simulink model "FCS-MPTC_10VVPTC_OEW_Simulink_file"  (R2024a)
settings: Solver=ode5  StartTime=0.0  StopTime=2  FixedStep=Ts  RelTol=1e-3
values from neighbouring files (symbols this model uses):
  J = 0.0148    [FivePhasePTCOEW.m]
  Ki = 0.0022    [FivePhasePTCOEW.m]
  Kp = 0.032    [FivePhasePTCOEW.m]
  kr = Lm/Lr    (= 0.941444444444)    [FivePhasePTCOEW.m]
  Lls = 6e-3    (= 0.006)    [FivePhasePTCOEW.m]
  Lm = 84.73e-3    (= 0.08473)    [FivePhasePTCOEW.m]
  p = 2    [FivePhasePTCOEW.m]
  r_sigma = Rs+kr^2*Rr    (= 2.3085710516)    [FivePhasePTCOEW.m]
  Rs = 1.05    [FivePhasePTCOEW.m]
  sf_nom = 0.2    [FivePhasePTCOEW.m]
  T_nom = 5    [FivePhasePTCOEW.m]
  t_sigma = sigma*Ls/r_sigma    (= 0.0044319243348)    [FivePhasePTCOEW.m]
  tr = Lr/Rr    (= 0.0633802816901)    [FivePhasePTCOEW.m]
  Ts = 5e-5    (= 5e-05)    [FivePhasePTCOEW.m]
  Vdc = 100    [FivePhasePTCOEW.m]
undefined symbols (not defined in the file or in its folder): DiscIntNeverNeededParam, j
libraries: simulink x2, simulink_extras x1, spspowerguiLib x1
settings Model: Creator=NARESH  LastModifiedBy=USER
settings ModelReferenceCC: EnableRefExpFcnMdlSchedulingChecks=on
settings RTWCC: GPUComputeCapability=3.5

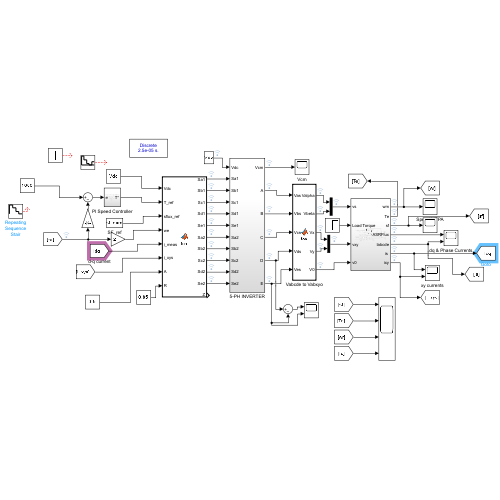
[thumbnail: Simulink's stored preview of the top-level diagram]
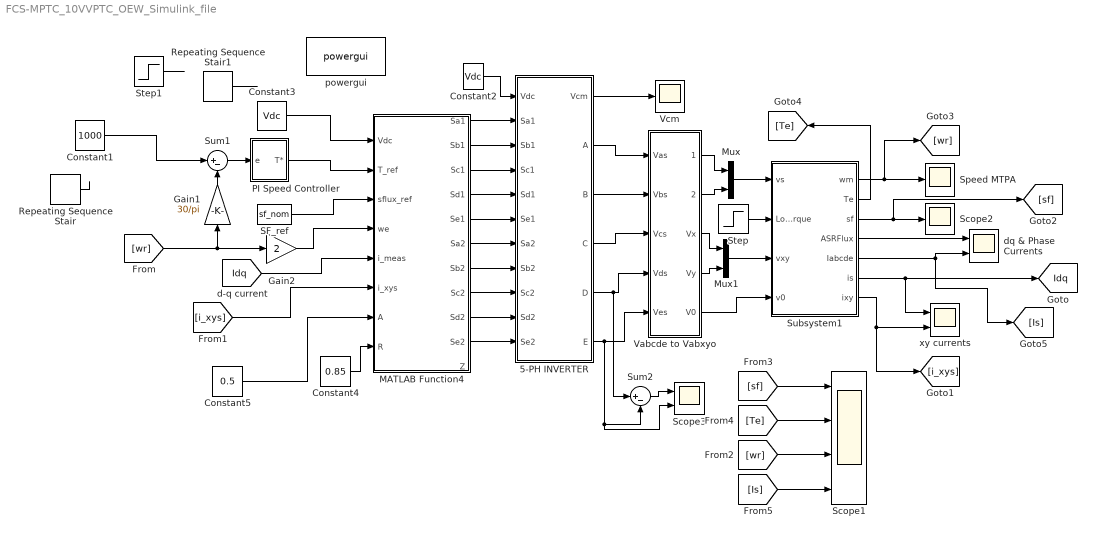
== system FCS-MPTC_10VVPTC_OEW_Simulink_file ==
  5-PH INVERTER : Subsystem
  Constant1 : Constant  Value=1000  SampleTime=Ts
  Constant2 : Constant  Value=Vdc  SampleTime=Ts
  Constant3 : Constant  Value=Vdc  SampleTime=Ts
  Constant4 : Constant  Value=0.85  SampleTime=Ts
  Constant5 : Constant  Value=0.5  SampleTime=Ts
  Gain1 : Gain  Gain=30/pi
  Gain2 : Gain  Gain=2
  MATLAB Function4 : MATLAB Function  TreatAsAtomicUnit=on
  Mux : Mux  Inputs=2
  Mux1 : Mux  Inputs=2
  PI Speed Controller : Subsystem
  Repeating Sequence Stair : simulink/Sources/Repeating Sequence Stair  OutValues=[1400 1000 500 200 ].'  tsamp=1.5  OutMin=[]  OutMax=[]  OutDataTypeStr=double  OutputDataTypeScalingMode=double  OutDataType=fixdt(0,8)  ConRadixGroup=Best Precision: Vector-wise  OutScaling=2^-12
  Repeating Sequence Stair1 : simulink/Sources/Repeating Sequence Stair  OutValues=[1400 800 200 0 500]  tsamp=1  OutMin=[]  OutMax=[]  OutDataTypeStr=double  OutputDataTypeScalingMode=double  OutDataType=fixdt(0,8)  ConRadixGroup=Best Precision: Vector-wise  OutScaling=2^-12
  SF_ref : Constant  Value=sf_nom  SampleTime=Ts
  Scope1 : Scope  NumInputPorts=4
  Scope2 : Scope
  Scope3 : Scope  NumInputPorts=2
  Speed MTPA : Scope
  Step : Step  After=0  SampleTime=0
  Step1 : Step  Before=400  After=-400  SampleTime=Ts
  Subsystem1 : Subsystem
  Sum1 : Sum  Inputs=|+-
  Sum2 : Sum  Inputs=|+-
  Vabcde to Vabxyo : MATLAB Function  TreatAsAtomicUnit=on
  Vcm : Scope
  dq & Phase Currents : Scope  NumInputPorts=2
  powergui : spspowerguiLib/powergui  Priority=1  SimulationMode=Discrete  SampleTime=Ts  frequency=60  Iterations=50  frequencyindice=60  Pbase=100e6  ErrMax=1e-4  UnitsV=kV  UnitsW=MW  buscounter=0  FunctionMessages=off  echomessages=off  EnableUseOfTLC=off  CurrentSourceSwitches=off  DisableSnubberDevices=off  DisableRonSwitches=off  DisableVfSwitches=off  DisplayEquations=off  AutomaticDiscreteSolvers=off  SolverType=Tustin/Backward Euler (TBE)  Interpol=off  ExternalGateDelay=off  methode=off  Ts=100  x0status=blocks  SPID=on  SwTol=0  HookPort=off  NonlinearTolerance=1e-4  nMaxIteration=100  ContinueOnMaxIteration=off  RestoreLinks=warning  ResistiveCurrentMeasurement=off  Frange=[0:2:500]  Ylog=off  Xlog=on  ShowGrid=off  save=off  variable=ZData  structure=0  ZoomFFT=off  StartTime=0.0  cycles=1  DisplayStyle=1  fundamental=60  FreqAxis=off  MaxFrequency=1000  frequencyindicesteady=1  RmsSteady=1  display=off
  xy currents : Scope  NumInputPorts=2
  tag scope: Idq=global
  wires:
  Subsystem1/3(sf) -> Scope2/1, [sf]
  5-PH INVERTER/2(A) -> Vabcde to Vabxyo/1(Vas)
  Subsystem1/7(ixy) -> xy currents/2, [i_xys]
  5-PH INVERTER/4(C) -> Vabcde to Vabxyo/3(Vcs)
  Subsystem1/1(wm) -> [wr], Speed MTPA/1
  5-PH INVERTER/3(B) -> Vabcde to Vabxyo/2(Vbs)
  Subsystem1/4(ASRFlux) -> dq & Phase Currents/1
  5-PH INVERTER/1(Vcm) -> Vcm/1
  Subsystem1/2(Te) -> [Te]
  Subsystem1/5(Iabcde) -> [Is], dq & Phase Currents/2
  Vabcde to Vabxyo/5(V0) -> Subsystem1/4(v0)
  Constant2/1 -> 5-PH INVERTER/1(Vdc)
  5-PH INVERTER/6(E) -> Scope3/2, Sum2/2, Vabcde to Vabxyo/5(Ves)
  Vabcde to Vabxyo/3(Vx) -> Mux1/1
  Vabcde to Vabxyo/1(Valpha) -> Mux/1
  Mux/1 -> Subsystem1/1(vs)
  Mux1/1 -> Subsystem1/3(vxy)
  Vabcde to Vabxyo/2(Vbeta) -> Mux/2
  5-PH INVERTER/5(D) -> Sum2/1, Vabcde to Vabxyo/4(Vds)
  Vabcde to Vabxyo/4(Vy) -> Mux1/2
  Subsystem1/6("is ") -> xy currents/1, [Idq]
  [wr] -> Scope1/3
  [sf] -> Scope1/1
  [Te] -> Scope1/2
  [Is] -> Scope1/4
  Sum2/1 -> Scope3/1
  Step/1 -> Subsystem1/2(Load Torque)
  MATLAB Function4/1(Sa1) -> 5-PH INVERTER/2(Sa1)
  MATLAB Function4/2(Sb1) -> 5-PH INVERTER/3(Sb1)
  MATLAB Function4/3(Sc1) -> 5-PH INVERTER/4(Sc1)
  MATLAB Function4/4(Sd1) -> 5-PH INVERTER/5(Sd1)
  MATLAB Function4/5(Se1) -> 5-PH INVERTER/6(Se1)
  MATLAB Function4/6(Sa2) -> 5-PH INVERTER/7(Sa2)
  MATLAB Function4/7(Sb2) -> 5-PH INVERTER/8(Sb2)
  MATLAB Function4/8(Sc2) -> 5-PH INVERTER/9(Sc2)
  MATLAB Function4/9(Sd2) -> 5-PH INVERTER/10(Sd2)
  MATLAB Function4/10(Se2) -> 5-PH INVERTER/11(Se2)
  Step1/1 -> ?
  [wr] -> Gain1/1, Gain2/1
  SF_ref/1 -> MATLAB Function4/3(sflux_ref)
  Constant4/1 -> MATLAB Function4/8(R)
  Sum1/1 -> PI Speed Controller/1(e)
  Constant3/1 -> MATLAB Function4/1(Vdc)
  Gain2/1 -> MATLAB Function4/4(we)
  Constant5/1 -> MATLAB Function4/7(A)
  Gain1/1 -> Sum1/2
  PI Speed Controller/1(T*) -> MATLAB Function4/2(T_ref)
  [i_xys] -> MATLAB Function4/6(i_xys)
  Repeating Sequence Stair1/1 -> ?
  [Idq] -> MATLAB Function4/5(i_meas)
  Constant1/1 -> Sum1/1
  Repeating Sequence Stair/1 -> ?

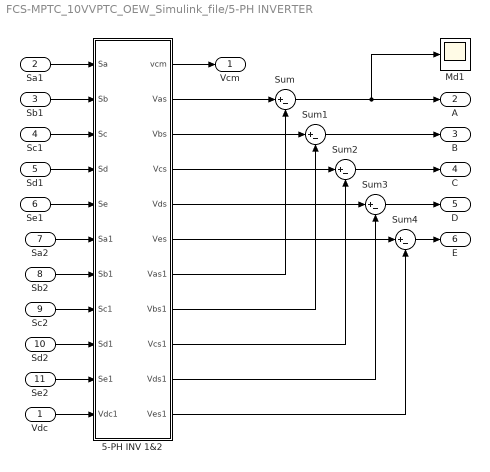
== system FCS-MPTC_10VVPTC_OEW_Simulink_file/5-PH INVERTER ==
  Vdc : Inport
  Sa1 : Inport  Port=2
  Sb1 : Inport  Port=3
  Sc1 : Inport  Port=4
  Sd1 : Inport  Port=5
  Se1 : Inport  Port=6
  Sa2 : Inport  Port=7
  Sb2 : Inport  Port=8
  Sc2 : Inport  Port=9
  Sd2 : Inport  Port=10
  Se2 : Inport  Port=11
  5-PH INV 1&2 : Subsystem
  Md1 : Scope
  Sum{,1..4} (5 alike) : Sum  Inputs=|+-
  Vcm : Outport
  A : Outport  Port=2
  B : Outport  Port=3
  C : Outport  Port=4
  D : Outport  Port=5
  E : Outport  Port=6
  wires:
  5-PH INV 1&2/6(Ves) -> Sum4/1
  5-PH INV 1&2/4(Vcs) -> Sum2/1
  5-PH INV 1&2/3(Vbs) -> Sum1/1
  5-PH INV 1&2/5(Vds) -> Sum3/1
  5-PH INV 1&2/2(Vas) -> Sum/1
  5-PH INV 1&2/11(Ves1) -> Sum4/2
  5-PH INV 1&2/9(Vcs1) -> Sum2/2
  5-PH INV 1&2/8(Vbs1) -> Sum1/2
  5-PH INV 1&2/7(Vas1) -> Sum/2
  Sum3/1 -> D/1
  Sum/1 -> Md1/1, A/1
  Sum1/1 -> B/1
  Sum2/1 -> C/1
  Sum4/1 -> E/1
  5-PH INV 1&2/10(Vds1) -> Sum3/2
  5-PH INV 1&2/1(vcm) -> Vcm/1
  Sa1/1 -> 5-PH INV 1&2/1(Sa)
  Sb1/1 -> 5-PH INV 1&2/2(Sb)
  Vdc/1 -> 5-PH INV 1&2/11(Vdc1)
  Sa2/1 -> 5-PH INV 1&2/6(Sa1)
  Sb2/1 -> 5-PH INV 1&2/7(Sb1)
  Sc2/1 -> 5-PH INV 1&2/8(Sc1)
  Sd2/1 -> 5-PH INV 1&2/9(Sd1)
  Se2/1 -> 5-PH INV 1&2/10(Se1)
  Se1/1 -> 5-PH INV 1&2/5(Se)
  Sd1/1 -> 5-PH INV 1&2/4(Sd)
  Sc1/1 -> 5-PH INV 1&2/3(Sc)

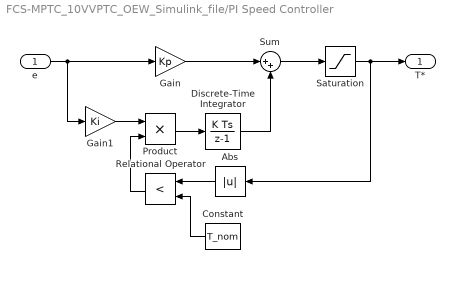
== system FCS-MPTC_10VVPTC_OEW_Simulink_file/PI Speed Controller ==
  e : Inport
  Abs : Abs  SaturateOnIntegerOverflow=off
  Constant : Constant  Value=T_nom
  Discrete-Time Integrator : DiscreteIntegrator  SampleTime=-1  ICPrevOutput=DiscIntNeverNeededParam  ICPrevScaledInput=DiscIntNeverNeededParam
  Gain : Gain  Gain=Kp
  Gain1 : Gain  Gain=Ki
  Product : Product
  Relational Operator : RelationalOperator  Operator=<  OutDataTypeStr=boolean  RndMeth=Simplest  InputSameDT=off
  Saturation : Saturate  UpperLimit=T_nom  LowerLimit=-T_nom
  Sum : Sum  Inputs=|++
  T* : Outport
  wires:
  Saturation/1 -> T*/1, Abs/1
  Sum/1 -> Saturation/1
  e/1 -> Gain1/1, Gain/1
  Product/1 -> Discrete-Time Integrator/1
  Gain1/1 -> Product/1
  Gain/1 -> Sum/1
  Discrete-Time Integrator/1 -> Sum/2
  Constant/1 -> Relational Operator/2
  Abs/1 -> Relational Operator/1
  Relational Operator/1 -> Product/2

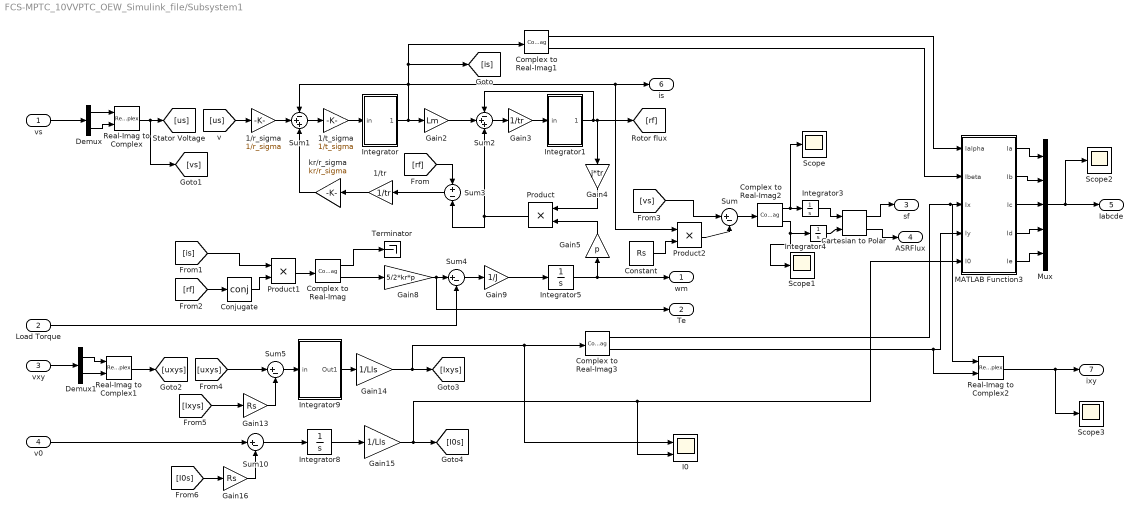
== system FCS-MPTC_10VVPTC_OEW_Simulink_file/Subsystem1 ==
  vs : Inport
  Load Torque : Inport  Port=2
  vxy : Inport  Port=3
  v0 : Inport  Port=4
  1/r_sigma : Gain  Gain=1/r_sigma
  1/t_sigma : Gain  Gain=1/t_sigma
  1/tr : Gain  Gain=1/tr
  Cartesian to Polar : simulink_extras/Transformations/Cartesian to Polar
  Complex to Real-Imag{,1..3} (4 alike) : ComplexToRealImag
  Conjugate : Math  Operator=conj  SignedPower=on  RndMeth=Zero
  Constant : Constant  Value=Rs  SampleTime=Ts
  Demux : Demux  Outputs=2
  Demux1 : Demux  Outputs=2
  Gain13 : Gain  Gain=Rs
  Gain14 : Gain  Gain=1/Lls
  Gain15 : Gain  Gain=1/Lls
  Gain16 : Gain  Gain=Rs
  Gain2 : Gain  Gain=Lm
  Gain3 : Gain  Gain=1/tr
  Gain4 : Gain  Gain=j*tr
  Gain5 : Gain  Gain=p
  Gain8 : Gain  Gain=5/2*kr*p
  Gain9 : Gain  Gain=1/J
  I0 : Scope  NumInputPorts=2
  Integrator : Subsystem
  Integrator1 : Subsystem
  Integrator{3..5,8} (4 alike) : Integrator
  Integrator9 : Subsystem
  MATLAB Function3 : MATLAB Function  TreatAsAtomicUnit=on
  Mux : Mux  Inputs=5
  Product : Product
  Product1 : Product
  Product2 : Product
  Real-Imag to Complex : RealImagToComplex
  Real-Imag to Complex1 : RealImagToComplex
  Real-Imag to Complex2 : RealImagToComplex
  Scope{,1..3} (4 alike) : Scope
  Sum{,4..5,10} (4 alike) : Sum  Inputs=|+-
  Sum1 : Sum  Inputs=-++
  Sum2 : Sum  Inputs=-++
  Sum3 : Sum  Inputs=+-
  Terminator : Terminator
  kr/r_sigma : Gain  Gain=kr/r_sigma
  wm : Outport
  Te : Outport  Port=2
  sf : Outport  Port=3
  ASRFlux : Outport  Port=4
  Iabcde : Outport  Port=5
  "is " : Outport  Port=6
  ixy : Outport  Port=7
  wires:
  Complex to Real-Imag3/1 -> Real-Imag to Complex2/1, MATLAB Function3/3(Ix)
  MATLAB Function3/5(Ie) -> Mux/5
  1/tr/1 -> kr/r_sigma/1
  Complex to Real-Imag2/2 -> Scope1/1, Integrator4/1
  Sum3/1 -> 1/tr/1
  Integrator1/1("Out1 ") -> Gain4/1, [rf], Sum2/1
  Integrator4/1 -> Cartesian to Polar/2
  MATLAB Function3/4(Id) -> Mux/4
  Gain16/1 -> Sum10/2
  [Ixys] -> Gain13/1
  Integrator/1("Out1 ") -> Gain2/1, Sum1/1, Complex to Real-Imag1/1, [is], "is "/1, Product2/1
  Gain15/1 -> I0/2, MATLAB Function3/5(I0), [I0s]
  Sum5/1 -> Integrator9/1(in)
  Gain14/1 -> I0/1, Complex to Real-Imag3/1, [Ixys]
  Demux1/1 -> Real-Imag to Complex1/1
  Demux1/2 -> Real-Imag to Complex1/2
  [us] -> 1/r_sigma/1
  [vs] -> Sum/1
  Demux/1 -> Real-Imag to Complex/1
  [uxys] -> Sum5/1
  Gain2/1 -> Sum2/2
  Complex to Real-Imag2/1 -> Scope/1, Integrator3/1
  Product2/1 -> Sum/2
  Cartesian to Polar/2 -> ASRFlux/1
  Product/1 -> Sum3/2, Sum2/3
  Real-Imag to Complex/1 -> [vs], [us]
  Constant/1 -> Product2/2
  Sum/1 -> Complex to Real-Imag2/1
  1/t_sigma/1 -> Integrator/1(in)
  Conjugate/1 -> Product1/2
  Real-Imag to Complex2/1 -> ixy/1, Scope3/1
  Cartesian to Polar/1 -> sf/1
  vs/1 -> Demux/1
  Gain3/1 -> Integrator1/1(in)
  Product1/1 -> Complex to Real-Imag/1
  Real-Imag to Complex1/1 -> [uxys]
  Gain13/1 -> Sum5/2
  Complex to Real-Imag1/1 -> MATLAB Function3/1(Ialpha)
  [is] -> Product1/1
  Gain8/1 -> Te/1, Sum4/1
  vxy/1 -> Demux1/1
  Sum1/1 -> 1/t_sigma/1
  Gain4/1 -> Product/1
  MATLAB Function3/2(Ib) -> Mux/2
  Mux/1 -> Iabcde/1, Scope2/1
  Complex to Real-Imag/2 -> Gain8/1
  Integrator9/1("Out1 ") -> Gain14/1
  Integrator8/1 -> Gain15/1
  Integrator5/1 -> wm/1, Gain5/1
  Gain5/1 -> Product/2
  Complex to Real-Imag/1 -> Terminator/1
  Complex to Real-Imag3/2 -> Real-Imag to Complex2/2, MATLAB Function3/4(Iy)
  Integrator3/1 -> Cartesian to Polar/1
  Gain9/1 -> Integrator5/1
  MATLAB Function3/1(Ia) -> Mux/1
  [rf] -> Sum3/1
  1/r_sigma/1 -> Sum1/2
  Demux/2 -> Real-Imag to Complex/2
  v0/1 -> Sum10/1
  Load Torque/1 -> Sum4/2
  Sum4/1 -> Gain9/1
  Complex to Real-Imag1/2 -> MATLAB Function3/2(Ibeta)
  Sum10/1 -> Integrator8/1
  [rf] -> Conjugate/1
  kr/r_sigma/1 -> Sum1/3
  MATLAB Function3/3(Ic) -> Mux/3
  Sum2/1 -> Gain3/1
  [I0s] -> Gain16/1

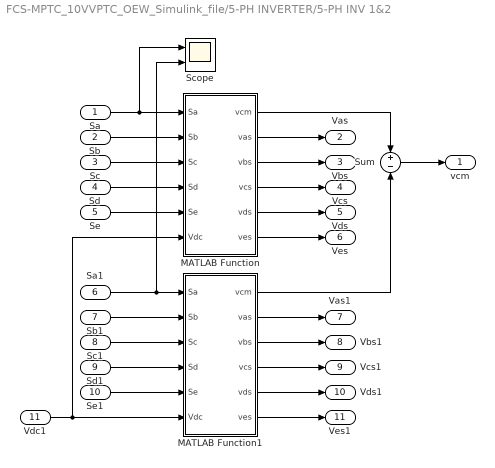
== system FCS-MPTC_10VVPTC_OEW_Simulink_file/5-PH INVERTER/5-PH INV 1&2 ==
  Sa : Inport
  Sb : Inport  Port=2
  Sc : Inport  Port=3
  Sd : Inport  Port=4
  Se : Inport  Port=5
  Sa1 : Inport  Port=6
  Sb1 : Inport  Port=7
  Sc1 : Inport  Port=8
  Sd1 : Inport  Port=9
  Se1 : Inport  Port=10
  Vdc1 : Inport  Port=11
  MATLAB Function : MATLAB Function  TreatAsAtomicUnit=on
  MATLAB Function1 : MATLAB Function  TreatAsAtomicUnit=on
  Scope : Scope  NumInputPorts=2
  Sum : Sum  Inputs=+-
  vcm : Outport
  Vas : Outport  Port=2
  Vbs : Outport  Port=3
  Vcs : Outport  Port=4
  Vds : Outport  Port=5
  Ves : Outport  Port=6
  Vas1 : Outport  Port=7
  Vbs1 : Outport  Port=8
  Vcs1 : Outport  Port=9
  Vds1 : Outport  Port=10
  Ves1 : Outport  Port=11
  wires:
  Sa/1 -> Scope/1, MATLAB Function/1(Sa)
  Sb/1 -> MATLAB Function/2(Sb)
  Sc/1 -> MATLAB Function/3(Sc)
  Sd/1 -> MATLAB Function/4(Sd)
  Se/1 -> MATLAB Function/5(Se)
  MATLAB Function/2(vas) -> Vas/1
  MATLAB Function/3(vbs) -> Vbs/1
  MATLAB Function/4(vcs) -> Vcs/1
  MATLAB Function/5(vds) -> Vds/1
  MATLAB Function/6(ves) -> Ves/1
  Sa1/1 -> Scope/2, MATLAB Function1/1(Sa)
  Sb1/1 -> MATLAB Function1/2(Sb)
  Sc1/1 -> MATLAB Function1/3(Sc)
  Sd1/1 -> MATLAB Function1/4(Sd)
  Se1/1 -> MATLAB Function1/5(Se)
  Vdc1/1 -> MATLAB Function/6(Vdc), MATLAB Function1/6(Vdc)
  MATLAB Function1/2(vas) -> Vas1/1
  MATLAB Function1/3(vbs) -> Vbs1/1
  MATLAB Function1/4(vcs) -> Vcs1/1
  MATLAB Function1/5(vds) -> Vds1/1
  MATLAB Function1/6(ves) -> Ves1/1
  MATLAB Function/1(vcm) -> Sum/1
  MATLAB Function1/1(vcm) -> Sum/2
  Sum/1 -> vcm/1

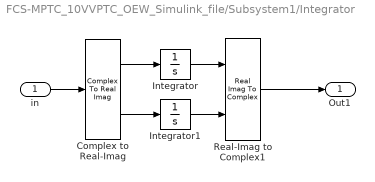
== system FCS-MPTC_10VVPTC_OEW_Simulink_file/Subsystem1/Integrator ==
  in : Inport
  Complex to Real-Imag : ComplexToRealImag
  Integrator : Integrator
  Integrator1 : Integrator
  Real-Imag to Complex1 : RealImagToComplex
  "Out1 " : Outport
  wires:
  Integrator/1 -> Real-Imag to Complex1/1
  in/1 -> Complex to Real-Imag/1
  Real-Imag to Complex1/1 -> "Out1 "/1
  Complex to Real-Imag/2 -> Integrator1/1
  Complex to Real-Imag/1 -> Integrator/1
  Integrator1/1 -> Real-Imag to Complex1/2

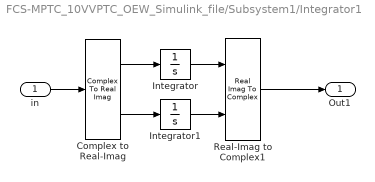
== system FCS-MPTC_10VVPTC_OEW_Simulink_file/Subsystem1/Integrator1 ==
  in : Inport
  Complex to Real-Imag : ComplexToRealImag
  Integrator : Integrator
  Integrator1 : Integrator
  Real-Imag to Complex1 : RealImagToComplex
  "Out1 " : Outport
  wires:
  Integrator1/1 -> Real-Imag to Complex1/2
  Complex to Real-Imag/1 -> Integrator/1
  Complex to Real-Imag/2 -> Integrator1/1
  Real-Imag to Complex1/1 -> "Out1 "/1
  in/1 -> Complex to Real-Imag/1
  Integrator/1 -> Real-Imag to Complex1/1

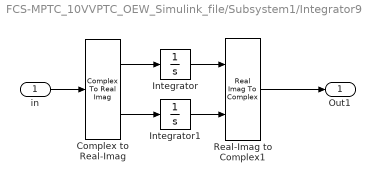
== system FCS-MPTC_10VVPTC_OEW_Simulink_file/Subsystem1/Integrator9 ==
  in : Inport
  Complex to Real-Imag : ComplexToRealImag
  Integrator : Integrator
  Integrator1 : Integrator
  Real-Imag to Complex1 : RealImagToComplex
  "Out1 " : Outport
  wires:
  Integrator/1 -> Real-Imag to Complex1/1
  in/1 -> Complex to Real-Imag/1
  Real-Imag to Complex1/1 -> "Out1 "/1
  Complex to Real-Imag/2 -> Integrator1/1
  Complex to Real-Imag/1 -> Integrator/1
  Integrator1/1 -> Real-Imag to Complex1/2

== matlab function FCS-MPTC_10VVPTC_OEW_Simulink_file/Subsystem1/MATLAB Function3 ==
  data: Ialpha input; Ia output; Ibeta input; Ix input; Iy input; I0 input; Ib output; Ic output; Id output; Ie output
function[Ia, Ib, Ic, Id, Ie] = fcn(Ialpha, Ibeta, Ix, Iy, I0)
Ia= 1*Ialpha+0*Ibeta+1*Ix-0*Iy+1*I0;
Ib= 0.3090*Ialpha+0.9511*Ibeta-0.8090*Ix-0.5878*Iy+1*I0;
Ic= -0.8090*Ialpha+0.5878*Ibeta+0.3090*Ix+0.9511*Iy+1*I0;
Id= -0.8090*Ialpha-0.5878*Ibeta+0.3090*Ix-0.9511*Iy+1*I0;
Ie= 0.3090*Ialpha-0.9511*Ibeta-0.8090*Ix+0.5878*Iy+1*I0;

== matlab function FCS-MPTC_10VVPTC_OEW_Simulink_file/5-PH INVERTER/5-PH INV 1&2/MATLAB Function1 ==
  data: vcm output; Sa input; vas output; Sb input; Sc input; Sd input; Se input; Vdc input; vbs output; vcs output; vds output; ves output
function [vcm,vas,vbs,vcs,vds,ves] = fcn(Sa,Sb,Sc,Sd,Se,Vdc)
vas=(Vdc/5)*(4*Sa-Sb-Sc-Sd-Se);
vbs=(Vdc/5)*(-Sa+4*Sb-Sc-Sd-Se);
vcs=(Vdc/5)*(-Sa-Sb+4*Sc-Sd-Se);
vds=(Vdc/5)*(-Sa-Sb-Sc+4*Sd-Se);
ves=(Vdc/5)*(-Sa-Sb-Sc-Sd+4*Se);
vcm=(Vdc/5)*(Sa+Sb+Sc+Sd+Se)-(Vdc/2);

== matlab function FCS-MPTC_10VVPTC_OEW_Simulink_file/Vabcde to Vabxyo ==
  data: Vas input; Valpha output; Vbs input; Vcs input; Vds input; Ves input; Vbeta output; Vx output; Vy output; V0 output
function[Valpha, Vbeta, Vx, Vy, V0] = fcn(Vas, Vbs, Vcs, Vds, Ves)
Valpha= (2/5)*(Vas+Vbs*cos(2*pi/5)+Vcs*cos(4*pi/5)+Vds*cos(6*pi/5)+Ves*cos(8*pi/5));
Vbeta=(2/5)*(0+Vbs*sin(2*pi/5)+Vcs*sin(4*pi/5)+Vds*sin(6*pi/5)+Ves*sin(8*pi/5));
Vx=(2/5)*(Vas+Vbs*cos(6*pi/5)+Vcs*cos(12*pi/5)+Vds*cos(18*pi/5)+Ves*cos(24*pi/5));
Vy=(2/5)*(0+Vbs*sin(6*pi/5)+Vcs*sin(12*pi/5)+Vds*sin(18*pi/5)+Ves*sin(24*pi/5));
V0=(2/5)*(0.5*Vas+0.5*Vbs+0.5*Vcs+0.5*Vds+0.5*Ves);

== matlab function FCS-MPTC_10VVPTC_OEW_Simulink_file/MATLAB Function4 ==
  settings: updateMethod=DISCRETE
  data: Sa1 output; Sb1 output; Sc1 output; Sd1 output; Se1 output; Vdc input; T_ref input; sflux_ref input; we input; Sa2 output; i_meas input; Sb2 output; Sc2 output; Sd2 output; Se2 output; i_xys input; A input; Z output; R input
function [Sa1,Sb1,Sc1,Sd1,Se1,Sa2,Sb2,Sc2,Sd2,Se2,Z] = fcn(Vdc,T_ref,sflux_ref,we,i_meas,i_xys,A,R)
% Variables defined in the parameters file
% Sampling time of the predictive algorithm [s]
 Ts = 10e-5;
 p = 2; % Pole pairs
 Lm = 84e-3; % Magnetizing inductance [H]
 Ls = 90e-3; % Stator inductance [H]
 Lr = 90e-3; % Rotor inductance [H]
 Lls = 6e-3;
 Rs = 1.05; % Stator resistance [Ohm]
 Rr = 1.42; % Rotor resistance [Ohm]
 sf_nom = 0.2; % Nominal stator flux [Wb]
 T_nom = 5; % Nominal torque [Nm]
% Auxiliary constants
 tr = Lr/Rr;
 sigma = 1-(((Lm)^2)/(Lr*Ls));
 kr = Lm/Lr;
 r_sigma = Rs+(kr^2)*Rr;
 t_sigma = sigma*Ls/r_sigma;
 % Weighting factor for the cost function of PTC
 lambda =R*T_nom/sf_nom;
 %%Vdc=100;
% Large voltage vectors of a-b plane
v25 = 0.6472*Vdc;
v24 = 0.5235*Vdc+1i*0.3804*Vdc;
v28 = 0.1999*Vdc+1i*0.6155*Vdc;
v12 = -0.1999*Vdc+1i*0.6155*Vdc;
v14 = -0.5235*Vdc+1i*0.3804*Vdc;
v6  = -0.6472*Vdc;
v7  = -0.5235*Vdc-1i*0.3804*Vdc;
v3  = -0.1999*Vdc-1i*0.6155*Vdc;
v19 = 0.1999*Vdc-1i*0.6155*Vdc;
v17 = 0.5235*Vdc-1i*0.3804*Vdc;
% Medimum voltage vectors of a-b plane
v16 = 0.4*Vdc;
v29 = 0.3236*Vdc+1i*0.2351*Vdc;
v8 = 0.1236*Vdc+1i*0.3804*Vdc;
v30 = -0.1236*Vdc+1i*0.3804*Vdc;
v4 = -0.3236*Vdc+1i*0.2351*Vdc;
v15 = -0.4*Vdc;
v2 = -0.3236*Vdc-1i*0.2351*Vdc;
v23 =-0.1236*Vdc-1i*0.3804*Vdc;
v1 = 0.1236*Vdc-1i*0.3804*Vdc;
v27 = 0.3236*Vdc-1i*0.2351*Vdc;
% Small voltage vectors of a-b plane
v9 = 0.2472*Vdc;
v26 = 0.1999*Vdc+1i*0.1453*Vdc;
v20 = 0.0763*Vdc+1i*0.2351*Vdc;
v13 = -0.0763*Vdc+1i*0.2351*Vdc;
v10 = -0.1999*Vdc+1i*0.1453*Vdc;
v22 = -0.2472*Vdc;
v5 = -0.1999*Vdc-1i*0.1453*Vdc;
v11 = -0.0763*Vdc-1i*0.2351*Vdc;
v18 = 0.0763*Vdc-1i*0.2351*Vdc;
v21 = 0.1999*Vdc-1i*0.1453*Vdc;
% Zero Voltage Vectors
 %v32 = 0;
 v31 = 0;
% Small Voltage vectors of x-y plane
v6x  = 0.2472*Vdc;
v19x = 0.19999*Vdc+1i*0.1453*Vdc;
v24x = 0.0763*Vdc+1i*0.2351*Vdc;
v14x = -0.0763*Vdc+1i*0.2351*Vdc;
v3x  = -0.19999*Vdc+1i*0.1453*Vdc;
v25x = -0.2472*Vdc;
v12x = -0.19999*Vdc-1i*0.1453*Vdc;
v7x  = -0.0763*Vdc-1i*0.2351*Vdc;
v17x = 0.0763*Vdc-1i*0.2351*Vdc;
v28x = 0.19999*Vdc-1i*0.1453*Vdc;
% Medimum Voltage vectors of x-y plane
v16x = 0.4*Vdc;
v30x = 0.3236*Vdc+1i*0.2351*Vdc;
v2x = 0.1236*Vdc+1i*0.3804*Vdc;
v27x = -0.1236*Vdc+1i*0.3804*Vdc;
v8x = -0.3236*Vdc+1i*0.2351*Vdc;
v15x = -0.4*Vdc;
v1x = -0.3236*Vdc-1i*0.2351*Vdc;
v29x = -0.1236*Vdc-1i*0.3804*Vdc;
v4x = 0.1236*Vdc-1i*0.3804*Vdc;
v23x = 0.3236*Vdc-1i*0.2351*Vdc;
% Large Voltage vectors of x-y plane
v22x = 0.6472*Vdc;
v18x = 0.5235*Vdc+1i*0.3804*Vdc;
v26x = 0.1999*Vdc+1i*0.6155*Vdc;
v10x = -0.1999*Vdc+1i*0.6155*Vdc;
v11x =-0.5235*Vdc+1i*0.3804*Vdc;
v9x = -0.6472*Vdc;
v13x = -0.5235*Vdc-1i*0.3804*Vdc;
v5x = -0.1999*Vdc-1i*0.6155*Vdc;
v21x = 0.1999*Vdc-1i*0.6155*Vdc;
v20x = 0.5235*Vdc-1i*0.3804*Vdc;
%Vector states
 % v_L1  =  [v31 v25 v16 v24 v29 v28 v8 v12 v30 v14 v4 v6 v15 v7 v2 v3 v23 v19 v1 v17 v27 v32];
 % vx_L1 = [v31 v25x v16x v24x v29x v28x v8x v12x v30x v14x v4x v6x v15x v7x v2x v3x v23x v19x v1x v17x v27x v32];
 % v_L2  =  [v32 v7 v2 v3 v23 v19 v1 v17 v27 v25 v16 v24 v29 v28 v8 v12 v30 v14 v4 v6 v15 v31];
 % vx_L2 = [v32 v7x v2x v3x v23x v19x v1x v17x v27x v25x v16x v24x v29x v28x v8x v12x v30x v14x v4x v6x v15x v31];
 v_L1  =  [v31 v25 v16 v9 v24 v29 v26 v28 v8 v20 v12 v30 v13 v14 v4 v10 v6 v15 v22 v7 v2 v5 v3 v23 v11 v19 v1 v18 v17 v27 v21 v31];
 vx_L1 = [v31 v25x v16x v9x v24x v29x v26x v28x v8x v20x v12x v30x v13x v14x v4x v10x v6x v15x v22x v7x v2x v5x v3x v23x v11x v19x v1x v18x v17x v27x v21x v31];
 v_L2  =  [v31 v7 v2 v5 v3 v23 v11 v19 v1 v18 v17 v27 v21 v25 v16 v9 v24 v29 v26 v28 v8 v20 v12 v30 v13 v14 v4 v10 v6 v15 v22 v31];
 vx_L2 = [v31 v7x v2x v5x v3x v23x v11x v19x v1x v18x v17x v27x v21x v25x v16x v9x v24x v29x v26x v28x v8x v20x v12x v30x v13x v14x v4x v10x v6x v15x v22x v31];
     v = (v_L1-v_L2);
    vx = (vx_L1-vx_L2);                                         
% Switching states
 % states1 = [1 1 1 1 1;1 1 0 0 1;1 0 0 0 0;1 1 0 0 0;1 1 1 0 1;1 1 1 0 0;0 1 0 0 0;0 1 1 0 0;1 1 1 1 0;0 1 1 1 0;0 0 1 0 0;0 0 1 1 0;0 1 1 1 1;0 0 1 1 1;0 0 0 1 0;0 0 0 1 1;1 0 1 1 1;1 0 0 1 1;0 0 0 0 1;1 0 0 0 1;1 1 0 1 1;0 0 0 0 0];
 % states2 = [1 1 1 1 1;0 0 1 1 1;0 0 0 1 0;0 0 0 1 1;1 0 1 1 1;1 0 0 1 1;0 0 0 0 1;1 0 0 0 1;1 1 0 1 1;1 1 0 0 1;1 0 0 0 0;1 1 0 0 0;1 1 1 0 1;1 1 1 0 0;0 1 0 0 0;0 1 1 0 0;1 1 1 1 0;0 1 1 1 0;0 0 1 0 0;0 0 1 1 0;0 1 1 1 1;0 0 0 0 0];
 states1 = [1 1 1 1 1;1 1 0 0 1;1 0 0 0 0;0 1 0 0 1;1 1 0 0 0;1 1 1 0 1;1 1 0 1 0;1 1 1 0 0;0 1 0 0 0;1 0 1 0 0;0 1 1 0 0;1 1 1 1 0;0 1 1 0 1;0 1 1 1 0;0 0 1 0 0;0 1 0 1 0;0 0 1 1 0;0 1 1 1 1;1 0 1 1 0;0 0 1 1 1;0 0 0 1 0;0 0 1 0 1;0 0 0 1 1;1 0 1 1 1;0 1 0 1 1;1 0 0 1 1;0 0 0 0 1;1 0 0 1 0;1 0 0 0 1;1 1 0 1 1;1 0 1 0 1;0 0 0 0 0];
 states2 = [1 1 1 1 1;0 0 1 1 1;0 0 0 1 0;0 0 1 0 1;0 0 0 1 1;1 0 1 1 1;0 1 0 1 1;1 0 0 1 1;0 0 0 0 1;1 0 0 1 0;1 0 0 0 1;1 1 0 1 1;1 1 0 0 1;1 1 0 0 1;1 0 0 0 0;0 1 0 0 1;1 1 0 0 0;1 1 1 0 1;1 1 0 1 0;1 1 1 0 0;0 1 0 0 0;1 0 1 0 0;0 1 1 0 0;1 1 1 1 0;0 1 1 0 1;0 1 1 1 0;0 0 1 0 0;0 1 0 1 0;0 0 1 1 0;0 1 1 1 1;1 0 1 1 0;0 0 0 0 0];
%global Ts Rs Lr Lm Ls p tr kr r_sigma t_sigma lambda v states
 persistent x_opt Fs 
 if isempty(x_opt), x_opt = 1; end
 if isempty(Fs), Fs = 0 + 1i*0; end
% Stator flux estimate
 Fs = Fs + Ts*(v(x_opt) - Rs*i_meas);
% Rotor flux estimate
 Fr = Lr/Lm*Fs+i_meas*(Lm-Lr*Ls/Lm);
% assumptions
 g_opt = 1e10;
 Z=x_opt;
 ismax = 7;
% For loop 
 for i = 1:32
% i-th voltage vector for current prediction
 v_o1 = v(i);
 v_o2 = vx(i); 
% Stator flux prediction at instant k+1
 Fsp1 = Fs + Ts*(v_o1) - Rs*Ts*i_meas;
% Stator current prediction at instant k+1
  Isp1 = (1+Ts/t_sigma)*i_meas+Ts/(t_sigma+Ts)*(1/r_sigma*(((kr/tr)-(kr*1i*we))*Fr+v_o1));
% Harmonic Current Prediction
  I_xysp1= i_xys+(1/Lls)*((Ts*v_o2)-(Rs*Ts*i_xys));
  i_xsp1 = real(I_xysp1);
  i_ysp1 = imag(I_xysp1);
% Current condition 
  if abs(Isp1)<ismax
     Imk1 = 0;
 else 
     Imk1 = inf;
 end
% Torque prediction at instant k+1
  Tp1 = 5/2*p*imag(conj(Fsp1)*Isp1);
%  Cost function
   g = abs(T_ref - Tp1)+ lambda*abs(sflux_ref-abs(Fsp1))+A*(abs(0-i_xsp1)+A*abs(0-i_ysp1))+Imk1;
 if (g<g_opt)
 g_opt =abs(g);
 x_opt = i;
 end
 end
  %**************************************
 % Optimization
 %[~, x_opt] = min(g);
 % Output switching states
 Sa1 = states1(x_opt,1);
 Sb1 = states1(x_opt,2);
 Sc1 = states1(x_opt,3);
 Sd1 = states1(x_opt,4);
 Se1 = states1(x_opt,5);
 Sa2 = states2(x_opt,1);
 Sb2 = states2(x_opt,2);
 Sc2 = states2(x_opt,3);
 Sd2 = states2(x_opt,4);
 Se2 = states2(x_opt,5);

== matlab function FCS-MPTC_10VVPTC_OEW_Simulink_file/5-PH INVERTER/5-PH INV 1&2/MATLAB Function ==
  data: vcm output; Sa input; vas output; Sb input; Sc input; Sd input; Se input; Vdc input; vbs output; vcs output; vds output; ves output
function [vcm,vas,vbs,vcs,vds,ves] = fcn(Sa,Sb,Sc,Sd,Se,Vdc)
vas=(Vdc/5)*(4*Sa-Sb-Sc-Sd-Se);
vbs=(Vdc/5)*(-Sa+4*Sb-Sc-Sd-Se);
vcs=(Vdc/5)*(-Sa-Sb+4*Sc-Sd-Se);
vds=(Vdc/5)*(-Sa-Sb-Sc+4*Sd-Se);
ves=(Vdc/5)*(-Sa-Sb-Sc-Sd+4*Se);
vcm=(Vdc/5)*(Sa+Sb+Sc+Sd+Se)-(Vdc/2);
